simulink model "SimulationModel"  (R2023b)
settings: Solver=VariableStepAuto  StartTime=0.0  StopTime=10.0  RelTol=1e-3
values from neighbouring files (symbols this model uses):
  Jt = Mp*(Lp^(2)) + Mw*(L^(2)) + Jp    (= 0.029004)    [Parametros.m]    (also in SimulationGraph.m; main.m)
  Mt = (Lp*Mp+L*Mw)*g    (= 1.338084)    [Parametros.m]    (also in SimulationGraph.m; main.m)
settings Model: Creator=joser  LastModifiedBy=joser

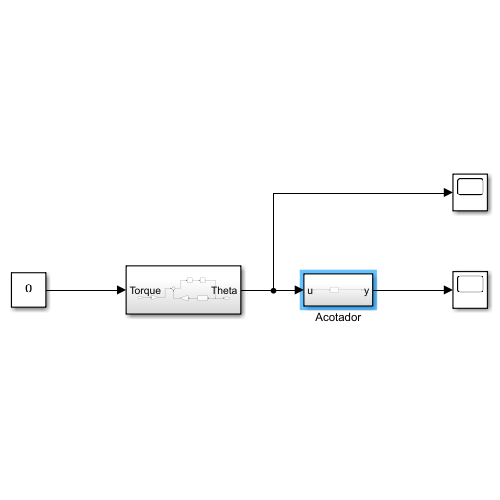
[thumbnail: Simulink's stored preview of the top-level diagram]
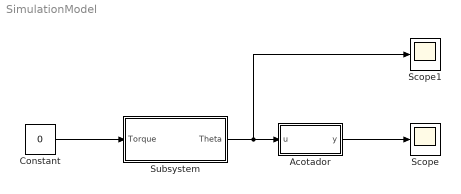
== system SimulationModel ==
  Acotador : Subsystem
  Constant : Constant  Value=0
  Scope : Scope
  Scope1 : Scope
  Subsystem : Subsystem
  wires:
  Subsystem/1(Theta) -> Scope1/1, Acotador/1(u)
  Constant/1 -> Subsystem/1(Torque)
  Acotador/1(y) -> Scope/1

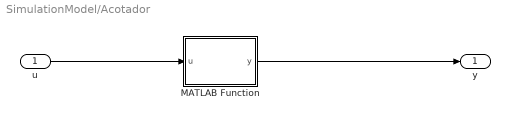
== system SimulationModel/Acotador ==
  u : Inport
  MATLAB Function : MATLAB Function  TreatAsAtomicUnit=on
  y : Outport
  wires:
  u/1 -> MATLAB Function/1(u)
  MATLAB Function/1(y) -> y/1

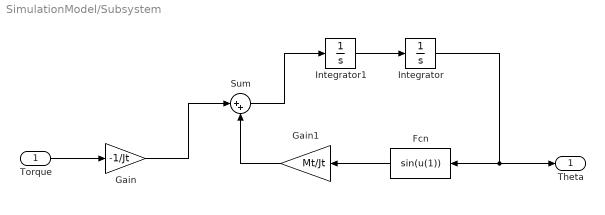
== system SimulationModel/Subsystem ==
  Torque : Inport
  Fcn : Fcn  Expr=sin(u(1))
  Gain : Gain  Gain=-1/Jt
  Gain1 : Gain  Gain=Mt/Jt
  Integrator : Integrator  InitialCondition=pi/2
  Integrator1 : Integrator
  Sum : Sum  Inputs=|++
  Theta : Outport
  wires:
  Torque/1 -> Gain/1
  Gain/1 -> Sum/1
  Gain1/1 -> Sum/2
  Integrator/1 -> Theta/1, Fcn/1
  Integrator1/1 -> Integrator/1
  Sum/1 -> Integrator1/1
  Fcn/1 -> Gain1/1

== matlab function SimulationModel/Acotador/MATLAB Function ==
  data: u input; y output
function y = fcn(u)

y = wrapToPi(u);
